simulink model "SimpleBEV"  (R2026a)
settings: Solver=VariableStepAuto
libraries: fl_lib x1, nesl_utility x1
settings Model: Creator=isaacito  LastModifiedBy=isaacito

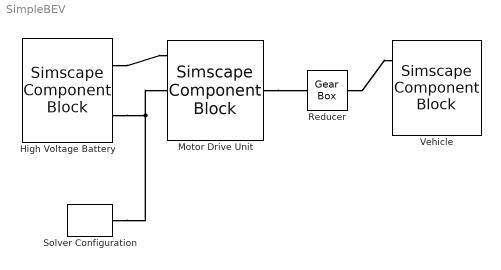
== system SimpleBEV ==
  High Voltage Battery : SimscapeComponentBlock  SourceFile=PrimitiveBattery  ComponentPath=PrimitiveBattery  ComponentVariants="[\"PrimitiveBattery\"]"  ComponentVariantNames="[\"PrimitiveBattery\"]"  ClassName=PrimitiveBattery  SchemaVersion=1  Vsys=340 V  Rin=0.01 Ohm
      settings: CopyFcn=simscape.sscblock.internal.componentBlockCallback(gcbh,'COPY')  PreCopyFcn=simscape.sscblock.internal.componentBlockCallback(gcbh,'PRECOPY')  PreDeleteFcn=simscape.sscblock.internal.componentBlockCallback(gcbh,'PREDELETE')
      mask Type: Primitive Battery
  Motor Drive Unit : SimscapeComponentBlock  SourceFile=IdealMotorDrive  ComponentPath=IdealMotorDrive  ComponentVariants="[\"IdealMotorDrive\"]"  ComponentVariantNames="[\"IdealMotorDrive\"]"  ClassName=IdealMotorDrive  SchemaVersion=1  torque_max=0.1 N*m  power_max=30 W  Tc=0.02 s  J_rotor=5e-6 kg*m^2  k_fric=1e-5 N*m*s/rad  speed0=0 rpm
      settings: CopyFcn=simscape.sscblock.internal.componentBlockCallback(gcbh,'COPY')  PreCopyFcn=simscape.sscblock.internal.componentBlockCallback(gcbh,'PRECOPY')  PreDeleteFcn=simscape.sscblock.internal.componentBlockCallback(gcbh,'PREDELETE')
      mask Type: Ideal Motor Drive Unit
  Reducer : fl_lib/Mechanical/Mechanisms/Gear Box  ratio=9.1  t_in_specify=off  t_in_priority=None  t_in=0 N*m  t_in_nominal_specify=off  t_in_nominal_value=1  t_in_nominal_unit=N*m  t_out_specify=off  t_out_priority=None  t_out=0 N*m  t_out_nominal_specify=off  t_out_nominal_value=1  t_out_nominal_unit=N*m
  Solver Configuration : nesl_utility/Solver Configuration  PhysicalDomain=network_engine_domain  SubClassName=solver  LeftPortType=input  RightPortType=generic  Tones=[]  Harmonics=[]  SimulateNoise=off  Profile=off  UseLocalSampling=off  EnableSwitchedLinearOptims=on  FrequencyDomain=off  UseCCode=off  RelTol=0.001  AbsTol=0.001  MinStep=1e-09  ToWorkspace=off  RevertToSquareIcSolve=off  NumHomotopyIterations=100  PhasorMode=off  PhasorModeNumHarmonics=1  ConsistencySolver=NEWTON_XTOL_AFTER_FTOL  CanonicalOrdering=CANONICAL  OptimizeIntermediates=OPTIMIZED  IndexReductionMethod=DerivativeReplacement  DoDC=off  ResidualTolerance=1e-09  ConsistencyTolSource=GLOBAL  ConsistencyAbsTol=0.001  ConsistencyRelTol=0.001  ConsistencyTolFactor=0.001  UseLocalSolver=off  LocalSolverChoice=NE_BACKWARD_EULER_ADVANCER  ResolveIndetEquations=on  FunctionEvalNumThread=1  LocalSolverSampleTime=0.001  DoFixedCost=off  MaxNonlinIter=3  MaxModeIter=2  ComputeImpulses=off  ImpulseIterations=2  LinearAlgebra=auto  LinearAlgebraNumThread=0  EquationFormulation=NE_TIME_EF  DelaysMemoryBudget=1024  AutomaticFiltering=on  FilteringTimeConstant=0.001  PartitionStorageMethod=AS_NEEDED  PartitionMemoryBudget=1024  PartitionMethod=ROBUST  MultibodyUseLocalSolver=off  MultibodyLocalSolverChoice=ODE1  MultibodyLocalSolverSampleTime=0.001
  Vehicle : SimscapeComponentBlock  SourceFile=IdealBEV  ComponentPath=IdealBEV  ComponentVariants="[\"IdealBEV\"]"  ComponentVariantNames="[\"IdealBEV\"]"  ClassName=IdealBEV  SchemaVersion=1  M_vehicle=2200 kg  R_tireroll=0.36 m  C_tireroll=0.0136  C_airdrag=0.31  A_front=2.3 m^2  air_density=1.184 kg/m^3  grav=9.81 m/s^2  V_1=0.1 km/hr  w_1=0.1 rpm  V_x_specify=off  V_x_priority=High  V_x=0 km/hr  V_x_nominal_specify=off  V_x_nominal_value=1  V_x_nominal_unit=km/hr  trq_specify=off  trq_priority=None  trq=0 N*m  trq_nominal_specify=off  trq_nominal_value=1  trq_nominal_unit=N*m  w_specify=off  w_priority=None  w=0 rpm  w_nominal_specify=off  w_nominal_value=1  w_nominal_unit=rpm
      settings: CopyFcn=simscape.sscblock.internal.componentBlockCallback(gcbh,'COPY')  PreCopyFcn=simscape.sscblock.internal.componentBlockCallback(gcbh,'PRECOPY')  PreDeleteFcn=simscape.sscblock.internal.componentBlockCallback(gcbh,'PREDELETE')
      mask Type: Ideal BEV
  connections:
  Reducer/RConn1 -- Vehicle/LConn1
  Motor Drive Unit/RConn1 -- Reducer/LConn1
  High Voltage Battery/RConn2 -- Solver Configuration/RConn1 -- Motor Drive Unit/LConn2
  High Voltage Battery/RConn1 -- Motor Drive Unit/LConn1
